simulink model "check_collision_with_bounding"  (R2018a)
settings: Solver=VariableStepAuto  StartTime=0.0  StopTime=120  FixedStep=0.01  MaxStep=.01  RelTol=1e-3
settings Model: Creator=U500304  LastModifiedBy=U500304
settings SolverCC: ZeroCrossAlgorithm=Adaptive
settings DataIOCC: SaveOutput=off  SaveTime=off
settings DebuggingCC: MaxConsecutiveZCsMsg=warning

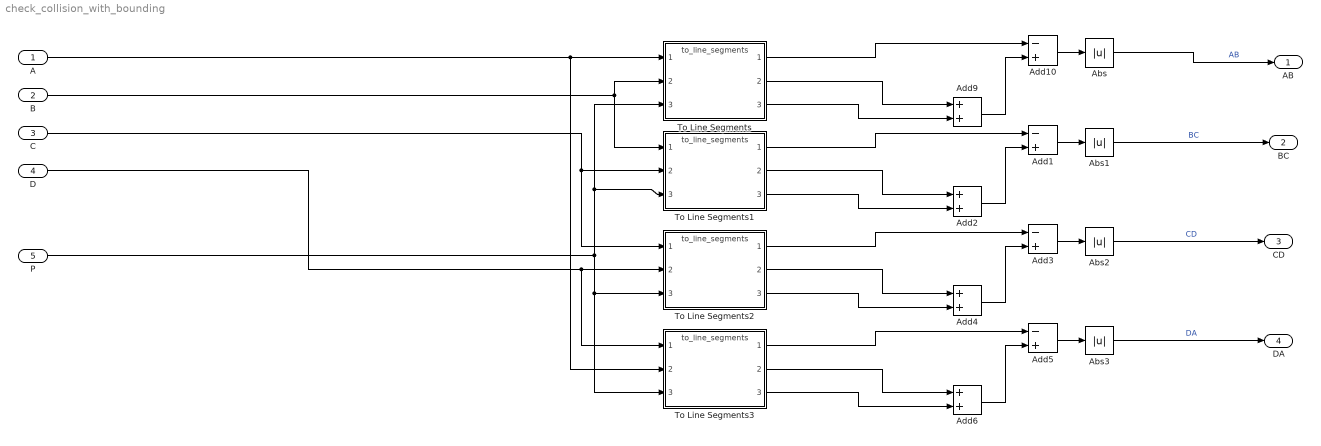
== system check_collision_with_bounding ==
  A : Inport  OutDataTypeStr=double  PortDimensions=2
  B : Inport  Port=2  OutDataTypeStr=double  PortDimensions=2
  C : Inport  Port=3  OutDataTypeStr=double  PortDimensions=2
  D : Inport  Port=4  OutDataTypeStr=double  PortDimensions=2
  P : Inport  Port=5  OutDataTypeStr=double  PortDimensions=2
  Abs{,1..3} (4 alike) : Abs
  Add{1,3,5,10} (4 alike) : Sum  Inputs=-+
  Add{2,4,6,9} (4 alike) : Sum
  To Line Segments{,1..3} (4 alike) : ModelReference  ModelNameDialog=to_line_segments.slx  SimulationMode=Normal  ModelReferenceVersion=1.639
  AB : Outport  OutDataTypeStr=double  PortDimensions=1  SampleTime=0
  BC : Outport  Port=2  OutDataTypeStr=double  PortDimensions=1  SampleTime=0
  CD : Outport  Port=3  OutDataTypeStr=double  PortDimensions=1  SampleTime=0
  DA : Outport  Port=4  OutDataTypeStr=double  PortDimensions=1  SampleTime=0
  wires:
  Add9/1 -> Add10/2
  To Line Segments/3 -> Add9/2
  To Line Segments3/2 -> Add6/1
  To Line Segments/1 -> Add10/1
  C/1 -> To Line Segments1/2, To Line Segments2/1
  To Line Segments2/3 -> Add4/2
  To Line Segments3/3 -> Add6/2
  To Line Segments/2 -> Add9/1
  To Line Segments1/1 -> Add1/1
  P/1 -> To Line Segments2/3, To Line Segments3/3, To Line Segments/3, To Line Segments1/3
  Add3/1 -> Abs2/1
  Add2/1 -> Add1/2
  Add10/1 -> Abs/1
  To Line Segments2/1 -> Add3/1
  To Line Segments2/2 -> Add4/1
  Add6/1 -> Add5/2
  A/1 -> To Line Segments/1, To Line Segments3/2
  B/1 -> To Line Segments1/1, To Line Segments/2
  Add5/1 -> Abs3/1
  D/1 -> To Line Segments2/2, To Line Segments3/1
  To Line Segments3/1 -> Add5/1
  To Line Segments1/2 -> Add2/1
  Abs3/1 -> DA/1  "DA"
  Add1/1 -> Abs1/1
  Add4/1 -> Add3/2
  Abs/1 -> AB/1  "AB"
  To Line Segments1/3 -> Add2/2
  Abs2/1 -> CD/1  "CD"
  Abs1/1 -> BC/1  "BC"
